simulink library "medusa5h1_stereo"  (R2022b)
settings: Solver=VariableStepAuto  StartTime=0.0  StopTime=10.0  RelTol=1e-3
values from neighbouring files (symbols this model uses):
  MedusaConfig = struct('BandSplitConfig', BandSplitConfig,                            'DRFDPConfig', DRFDPConfig,                            'FRFDPConfig', FRFDPConfig,                            'SurroundConfig', SurroundConfig,                            'MSConfig', MSConfig,                            'PremixConfig', PremixConfig.Stereo,                            'PremixTune', PremixTune.Stereo,               ...(+1303 chars)    [medusa5h1_init.m]
undefined symbols (not defined in the file or in its folder): Config, MedusaBTC, Row, VLSConfig
libraries: TuneVar x25, MedusaDelays x19, FeaturePath x15, RTC x6, MedusaCaeEnable x4, MedusaDrHoligramEq x4, TOP x4, BassManager x2, StateVar x2, TrebleBoost x2, dspstat3 x2, MedusaBandSplit x2
(part 1 of 2)
settings Model: Creator=ud1041536  LastModifiedBy=mp55777
settings SolverCC: AlgebraicLoopSolver=TrustRegion
settings DebuggingCC: UnconnectedInputMsg=warning  UnconnectedOutputMsg=warning  UnconnectedLineMsg=warning  SFMachineParentedDataDiag=warning  ArithmeticOperatorsInVariantConditions=warning
settings ModelReferenceCC: EnableRefExpFcnMdlSchedulingChecks=on
settings SFSimCC: CustomCodeUndefinedFunction=UseInterfaceOnly

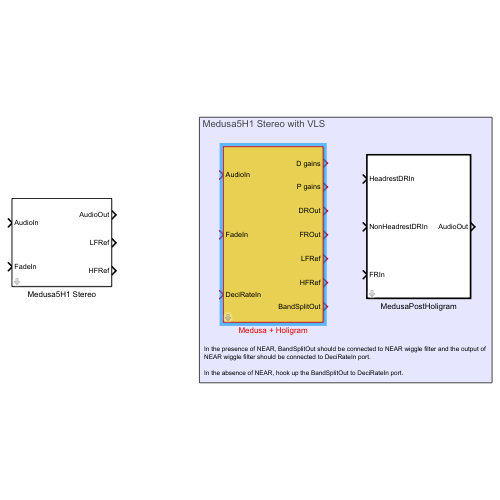
[thumbnail: Simulink's stored preview of the top-level diagram]
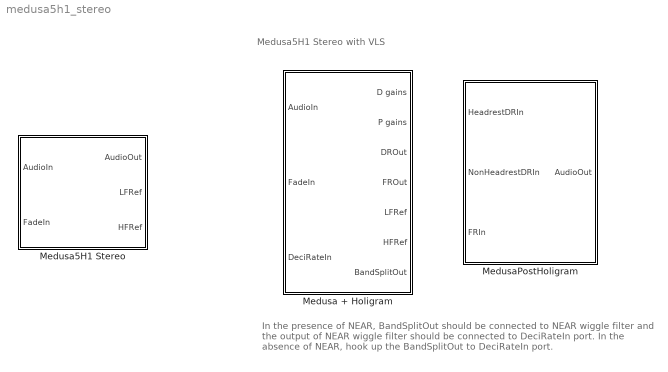
== system medusa5h1_stereo ==
  note: Medusa5H1 Stereo with VLS
  note: In the presence of NEAR, BandSplitOut should be connected to NEAR wiggle filter and the output of
      | NEAR wiggle filter should be connected to DeciRateIn port.
      |
      | In the absence of NEAR, hook up the BandSplitOut to DeciRateIn port.
  Medusa + Holigram : Subsystem  mask{config=MedusaConfig, ConfigBTC=MedusaBTC, vlsConfigStruct=VLSConfig}
      mask prompts: config "Medusa config struct name:"; ConfigBTC "Medusa BTC config struct name:"; vlsConfigStruct "VLS config struct name:"
      mask init:
      | tailCompEQ = config.tailCompEQ;
      | HRDelayConfig = vlsConfigStruct.HeadrestDelayConfig;
      settings: LibrarySourceBlock=medusa5h1_stereo/Medusa + Holigram
  Medusa5H1 Stereo : Subsystem  mask{config=MedusaConfig}
      mask prompts: config "Config struct name:"
      mask init:
      | tailCompEQ = config.tailCompEQ;
      | % delayConfig = config.DelayConfig;
      | 
      | % % Set 2 Medusa parts to be atomic if in Indirect Addressing Mode
      | % isIndirect = CoreIndexMask.IsIndirectAddressing(gcbh);
      | % if isIndirect
      | %     atomicSetting = 'on';
      | % else
      | %     atomicSetting = 'off';
      | % end
      | % p1Name = MaskUtil.SubBlockName(gcbh, 'Medusa5H1 Part 1');
      | % p2Name = MaskUtil.SubBlockName(gcbh, 'Medusa5H1 Part 2');
      | % 
      | % if -1 ~= (getSimulinkBlockHandle(p1Name))
      | %     MaskUtil.safe_setparam(p1Name, 'TreatAsAtomicUnit', atomicSetting);
      | % end
      | % 
      | % if -1 ~= (getSimulinkBlockHandle(p2Name))
      | %     MaskUtil.safe_setparam(p2Name, 'TreatAsAtomicUnit', atomicSetting);
      | % end
  MedusaPostHoligram : Subsystem  TreatAsAtomicUnit=on  mask{config=MedusaConfig}
      mask prompts: config "Config struct name:"
      settings: RTWSystemCode=Nonreusable function  RTWFcnNameOpts=Use subsystem name  RTWFileNameOpts=Use subsystem name  FunctionWithSeparateData=on

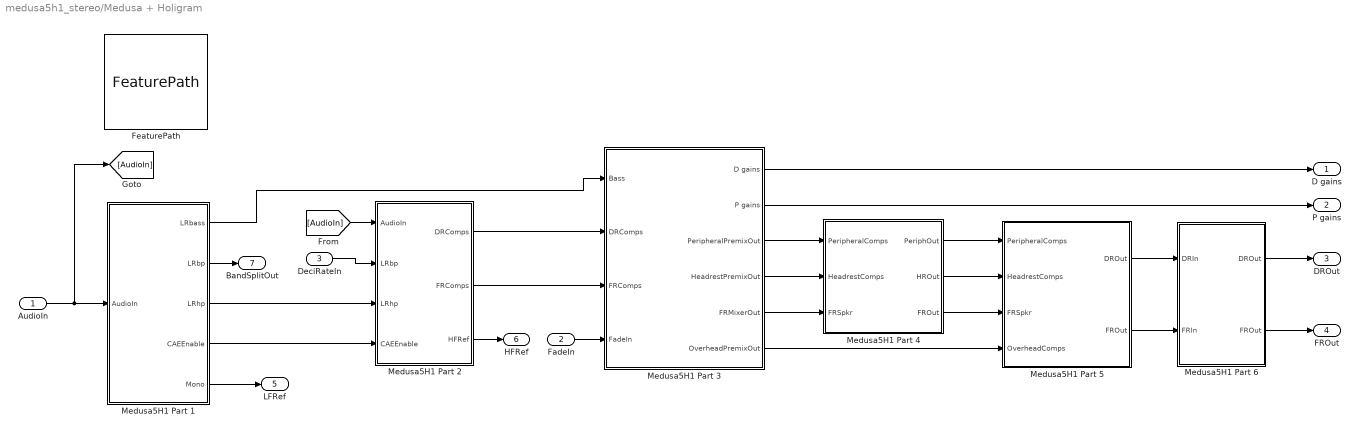
== system medusa5h1_stereo/Medusa + Holigram ==
  AudioIn : Inport
  FadeIn : Inport  Port=2  OutDataTypeStr=single
  DeciRateIn : Inport  Port=3
  FeaturePath : FeaturePath/FeaturePath  FeatureName=Medusa  IsGroup=off  GroupNumber=-1  IsModule=off  TriggerInit=[90 69 205 176]
      settings: SourceProductName=Bose Talaria
  Medusa5H1 Part 1 : Subsystem  TreatAsAtomicUnit=on
      settings: RTWSystemCode=Nonreusable function
  Medusa5H1 Part 2 : Subsystem  TreatAsAtomicUnit=on
      settings: RTWSystemCode=Nonreusable function
  Medusa5H1 Part 3 : Subsystem  TreatAsAtomicUnit=on
      settings: RTWSystemCode=Nonreusable function  FunctionWithSeparateData=on
  Medusa5H1 Part 4 : Subsystem  TreatAsAtomicUnit=on  RTWFcnName=MedusaHoligram  RTWFileName=MedusaHoligram
      settings: RTWSystemCode=Nonreusable function  FunctionWithSeparateData=on
  Medusa5H1 Part 5 : Subsystem  TreatAsAtomicUnit=on
      settings: RTWSystemCode=Nonreusable function  FunctionWithSeparateData=on
  Medusa5H1 Part 6 : Subsystem  TreatAsAtomicUnit=on
      settings: RTWSystemCode=Nonreusable function  FunctionWithSeparateData=on
  D gains : Outport
  P gains : Outport  Port=2
  DROut : Outport  Port=3
  FROut : Outport  Port=4
  LFRef : Outport  Port=5  VectorParamsAs1DForOutWhenUnconnected=off
  HFRef : Outport  Port=6  VectorParamsAs1DForOutWhenUnconnected=off
  BandSplitOut : Outport  Port=7
  wires:
  Medusa5H1 Part 2/2(FRComps) -> Medusa5H1 Part 3/3(FRComps)
  Medusa5H1 Part 2/1(DRComps) -> Medusa5H1 Part 3/2(DRComps)
  FadeIn/1 -> Medusa5H1 Part 3/4(FadeIn)
  AudioIn/1 -> [AudioIn], Medusa5H1 Part 1/1(AudioIn)
  Medusa5H1 Part 1/5(Mono) -> LFRef/1
  Medusa5H1 Part 1/3(LRhp) -> Medusa5H1 Part 2/3(LRhp)
  [AudioIn] -> Medusa5H1 Part 2/1(AudioIn)
  Medusa5H1 Part 1/1(LRbass) -> Medusa5H1 Part 3/1(Bass)
  Medusa5H1 Part 3/2(P gains) -> P gains/1
  Medusa5H1 Part 3/1(D gains) -> D gains/1
  Medusa5H1 Part 6/1(DROut) -> DROut/1
  Medusa5H1 Part 6/2(FROut) -> FROut/1
  Medusa5H1 Part 2/3(HFRef) -> HFRef/1
  Medusa5H1 Part 1/4(CAEEnable) -> Medusa5H1 Part 2/4(CAEEnable)
  Medusa5H1 Part 3/3(PeripheralPremixOut) -> Medusa5H1 Part 4/1(PeripheralComps)
  Medusa5H1 Part 3/4(HeadrestPremixOut) -> Medusa5H1 Part 4/2(HeadrestComps)
  Medusa5H1 Part 3/5(FRMixerOut) -> Medusa5H1 Part 4/3(FRSpkr)
  Medusa5H1 Part 1/2(LRbp) -> BandSplitOut/1
  DeciRateIn/1 -> Medusa5H1 Part 2/2(LRbp)
  Medusa5H1 Part 4/1(PeriphOut) -> Medusa5H1 Part 5/1(PeripheralComps)
  Medusa5H1 Part 4/2(HROut) -> Medusa5H1 Part 5/2(HeadrestComps)
  Medusa5H1 Part 4/3(FROut) -> Medusa5H1 Part 5/3(FRSpkr)
  Medusa5H1 Part 5/1(DROut) -> Medusa5H1 Part 6/1(DRIn)
  Medusa5H1 Part 5/2(FROut) -> Medusa5H1 Part 6/2(FRIn)
  Medusa5H1 Part 3/6(OverheadPremixOut) -> Medusa5H1 Part 5/4(OverheadComps)

== system medusa5h1_stereo/Medusa5H1 Stereo ==
  AudioIn : Inport
  FadeIn : Inport  Port=2  OutDataTypeStr=single
  FeaturePath : FeaturePath/FeaturePath  FeatureName=Medusa  IsGroup=off  GroupNumber=-1  IsModule=off  TriggerInit=[615 344 730 451]
      settings: SourceProductName=Bose Talaria
  Medusa5H1 Part 1 : Subsystem  TreatAsAtomicUnit=on
      settings: RTWSystemCode=Nonreusable function
  Medusa5H1 Part 2 : Subsystem  TreatAsAtomicUnit=on
      settings: RTWSystemCode=Nonreusable function
  Medusa5H1 Part 3 : Subsystem  TreatAsAtomicUnit=on
      settings: RTWSystemCode=Nonreusable function  FunctionWithSeparateData=on
  Medusa5H1 Part 4 : Subsystem  TreatAsAtomicUnit=on
      settings: RTWSystemCode=Nonreusable function  FunctionWithSeparateData=on
  AudioOut : Outport  VectorParamsAs1DForOutWhenUnconnected=off
  LFRef : Outport  Port=2  VectorParamsAs1DForOutWhenUnconnected=off
  HFRef : Outport  Port=3  VectorParamsAs1DForOutWhenUnconnected=off
  wires:
  Medusa5H1 Part 1/1(LRbass) -> Medusa5H1 Part 3/1(Bass)
  Medusa5H1 Part 2/1(DRComps) -> Medusa5H1 Part 3/2(DRComps)
  Medusa5H1 Part 2/2(FRComps) -> Medusa5H1 Part 3/3(FRComps)
  FadeIn/1 -> Medusa5H1 Part 3/4(FadeIn)
  Medusa5H1 Part 1/2(LRbp) -> Medusa5H1 Part 2/2(LRbp)
  Medusa5H1 Part 1/3(LRhp) -> Medusa5H1 Part 2/3(LRhp)
  AudioIn/1 -> [AudioIn], Medusa5H1 Part 1/1(AudioIn)
  [AudioIn] -> Medusa5H1 Part 2/1(AudioIn)
  Medusa5H1 Part 4/1(Out) -> AudioOut/1
  Medusa5H1 Part 3/1(PeripheralPremixOut) -> Medusa5H1 Part 4/1(PeripheralPremixComps)
  Medusa5H1 Part 3/3(FRMixerOut) -> Medusa5H1 Part 4/3(FRSpkrs)
  Medusa5H1 Part 1/5(Mono) -> LFRef/1
  Medusa5H1 Part 2/3(HFRef) -> HFRef/1
  Medusa5H1 Part 1/4(CAEEnable) -> Medusa5H1 Part 2/4(CAEEnable)
  Medusa5H1 Part 3/2(OverheadPremixOut) -> Medusa5H1 Part 4/2(OverheadPremixComps)

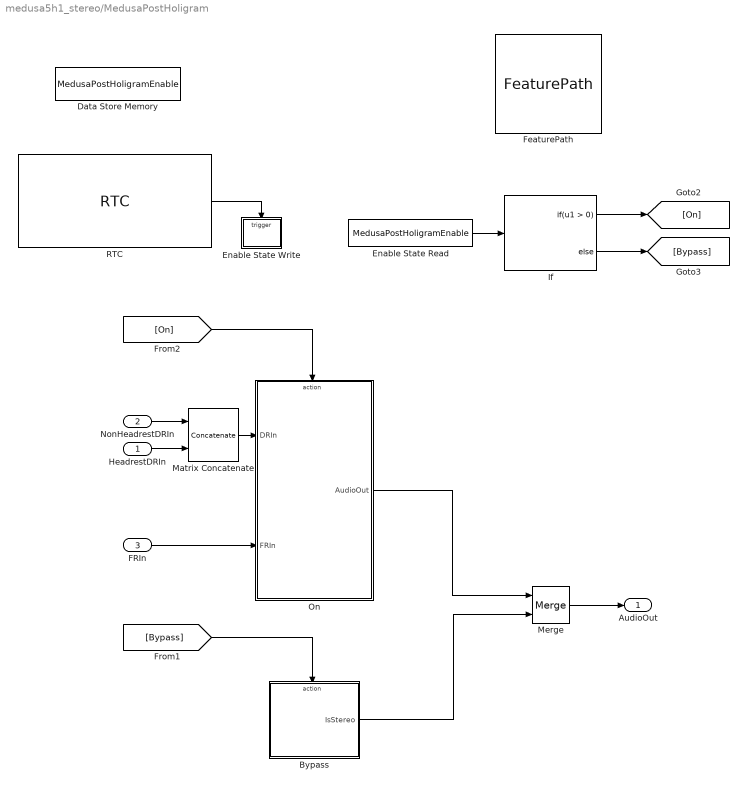
== system medusa5h1_stereo/MedusaPostHoligram ==
  HeadrestDRIn : Inport
  NonHeadrestDRIn : Inport  Port=2
  FRIn : Inport  Port=3
  Bypass : Subsystem
  Data Store Memory : DataStoreMemory  DataStoreName=MedusaPostHoligramEnable  ReadBeforeWriteMsg=warning  WriteAfterWriteMsg=warning  WriteAfterReadMsg=warning  InitialValue=1  ShowAdditionalParam=off  OutDataTypeStr=uint32
  Enable State Read : DataStoreRead  DataStoreName=MedusaPostHoligramEnable  IndexOptions=Index vector (dialog)  Indices=1  OutputSizes=1
  Enable State Write : Subsystem
  FeaturePath : FeaturePath/FeaturePath  FeatureName=Medusa  IsGroup=off  GroupNumber=-1  IsModule=off  TriggerInit=[810 309 925 416]
      settings: SourceProductName=Bose Talaria
  If : If
  Matrix Concatenate : Concatenate  Mode=Multidimensional array  ConcatenateDimension=2
  Merge : Merge  InitialOutput=MedusaConfig.outputDefault
  On : Subsystem
  RTC : RTC/RTC  REQ_Priority=RTC_Mask.NormalPriority  RequestAtInit=off  EnableRequest=on  REQElemType1=int32  REQElemWidth1=1  REQElemInitial1=[]  REQElemType2=uint32  REQElemWidth2=1  REQElemInitial2=[]  REQElemType3=uint32  REQElemWidth3=1  REQElemInitial3=[]  REQElemType4=uint32  REQElemWidth4=1  REQElemInitial4=[]  REQElemType5=uint32  REQElemWidth5=1  REQElemInitial5=[]  REQElemType6=uint32  REQElemWidth6=1  REQElemInitial6=[]  REQElemType7=uint32  REQElemWidth7=1  REQElemInitial7=[]  REQElemType8=uint32  REQElemWidth8=1  REQElemInitial8=[]  REQElemType9=uint32  REQElemWidth9=1  REQElemInitial9=[]  REQElemType10=uint32  REQElemWidth10=1  REQElemInitial10=[]  EnableResponse=on  EnableRSP_StatusIn=off  RSPElemType1=uint32  RSPElemWidth1=1  RSPElemType2=uint32  RSPElemWidth2=1  RSPElemType3=uint32  RSPElemWidth3=1  RSPElemType4=uint32  RSPElemWidth4=1  RSPElemType5=uint32  RSPElemWidth5=1  RSPElemType6=uint32  RSPElemWidth6=1  RSPElemType7=uint32  RSPElemWidth7=1  RSPElemType8=uint32  RSPElemWidth8=1  RSPElemType9=uint32  RSPElemWidth9=1  RSPElemType10=uint32  RSPElemWidth10=1  EnableNotification=off  EnableNTF_PrepTrig=off  NTFElemType1=uint32  NTFElemWidth1=1  NTFElemType2=uint32  NTFElemWidth2=1  NTFElemType3=uint32  NTFElemWidth3=1  NTFElemType4=uint32  NTFElemWidth4=1  NTFElemType5=uint32  NTFElemWidth5=1  NTFElemType6=uint32  NTFElemWidth6=1  NTFElemType7=uint32  NTFElemWidth7=1  NTFElemType8=uint32  NTFElemWidth8=1  NTFElemType9=uint32  NTFElemWidth9=1  NTFElemType10=uint32  NTFElemWidth10=1  MaskMessageName=PostHoligramDisable
      settings: SourceProductName=Bose Talaria
  AudioOut : Outport  VectorParamsAs1DForOutWhenUnconnected=off
  wires:
  FRIn/1 -> On/2(FRIn)
  [Bypass] -> Bypass/Action
  Bypass/1(IsStereo) -> Merge/2
  On/1(AudioOut) -> Merge/1
  Merge/1 -> AudioOut/1
  If/1 -> [On]
  If/2 -> [Bypass]
  Enable State Read/1 -> If/1
  [On] -> On/Action
  RTC/1 -> Enable State Write/Trigger
  Matrix Concatenate/1 -> On/1(DRIn)
  NonHeadrestDRIn/1 -> Matrix Concatenate/1
  HeadrestDRIn/1 -> Matrix Concatenate/2

== system medusa5h1_stereo/Medusa + Holigram/Medusa5H1 Part 1 ==
  AudioIn : Inport
  Bass Manager Stereo : BassManager/MedusaBassManager  Config=ConfigBTC.BassManager
  CAE Treble Boost : Subsystem  Variant=on
  Mean : dspstat3/Mean  run=off  InputProcessing=Columns as channels (frame based)  reset_popup=None  directionMode=Each row  dimension=1  roiEnable=off  roiType=Rectangles  roiPortion=Entire ROI  roiOutput=Individual statistics for each ROI  roiFlag=off  roundingMode=Floor  overflowMode=off  outputDataTypeStr=Inherit: Same as accumulator  outputMin=[]  outputMax=[]  outputLastDataTypeStr=Inherit: Same as accumulator
  Medusa Band Split Stereo : MedusaBandSplit/Medusa Band Split Stereo  configStruct=config.BandSplitConfig
  Partition : FeaturePath/Partition  PartitionNumber=2  TriggerInit=[375 -99 420 -31]
      settings: SourceProductName=Bose Talaria
  Terminator : Terminator
  TuneVar : TuneVar/TuneVar  Description=|  TuneName=SurroundOn  SpecifyMaxSize=off  VariableDim=1 (Row)  MaxSize=[1 1]  TunabilityNumber=1  MinValue=[]  MaxValue=[]  TriggerInit=[235 97 315 133]  MaskValue=ConfigBTC.TuneVarBmSurroundOn
      | General surround control parameter
      | STEREO_MODE = 0
      | SURROUND_PASSTHRU_MODE = 1
      | MEDUSA_2_CHANNEL_MODE = 2
      | MEDUSA_5_1_MODE = 3
      settings: SourceProductName=Bose Talaria
  LRbass : Outport  VectorParamsAs1DForOutWhenUnconnected=off
  LRbp : Outport  Port=2  VectorParamsAs1DForOutWhenUnconnected=off
  LRhp : Outport  Port=3  VectorParamsAs1DForOutWhenUnconnected=off
  CAEEnable : Outport  Port=4
  Mono : Outport  Port=5  VectorParamsAs1DForOutWhenUnconnected=off
  wires:
  Medusa Band Split Stereo/2 -> LRhp/1  "LRtreble"
  Bass Manager Stereo/1 -> LRbass/1  "Lbass, Rbass"
  Medusa Band Split Stereo/1 -> LRbp/1  "LRbp"
  Bass Manager Stereo/2 -> Medusa Band Split Stereo/1
  CAE Treble Boost/1(Out) -> Mean/1, Bass Manager Stereo/1  "L, R"
  Mean/1 -> Mono/1
  AudioIn/1 -> CAE Treble Boost/1(AudioIn)  "L, R"
  CAE Treble Boost/2(CAEEnable) -> CAEEnable/1
  Bass Manager Stereo/3 -> Terminator/1
  TuneVar/1 -> Bass Manager Stereo/2  "SurroundOn"

== system medusa5h1_stereo/Medusa + Holigram/Medusa5H1 Part 2 ==
  AudioIn : Inport  OutDataTypeStr=single
  LRbp : Inport  Port=2
  LRhp : Inport  Port=3
  CAEEnable : Inport  Port=4
  Alignment Delay : Subsystem  TreatAsAtomicUnit=on
      settings: RTWSystemCode=Nonreusable function  FunctionWithSeparateData=on
  Decimated-Rate FDP : MedusaFdp/MedusaFdp  Config=ConfigBTC.DeciRateFdp
  Full-Rate FDP : MedusaFdp/MedusaFdp  Config=ConfigBTC.FullRateFdp
  Mono Detector : MonoDetector/MedusaMonoDetector  Config=ConfigBTC.MonoDetector
  Partition : FeaturePath/Partition  PartitionNumber=3  TriggerInit=[825 236 870 304]
      settings: SourceProductName=Bose Talaria
  SPUM Decay Estimate : MedusaSPUMDecayEst/SPUM Decay Estimate  configStruct=config.FRFDPConfig
  Selector : Selector  NumberOfDimensions=2  InputPortWidth=3  IndexOptions=Select all,Index vector (dialog)  Indices=[1 3],[1,2]  OutputSizes=1,1
  Selector1 : Selector  NumberOfDimensions=2  InputPortWidth=3  IndexOptions=Select all,Index vector (dialog)  Indices=[1 3],[1 2 3 5]  OutputSizes=1,1
  DRComps : Outport  VectorParamsAs1DForOutWhenUnconnected=off
  FRComps : Outport  Port=2  VectorParamsAs1DForOutWhenUnconnected=off
  HFRef : Outport  Port=3
  wires:
  Decimated-Rate FDP/1 -> DRComps/1  "Lo, Ro, Ls, Rs, Limp, Ltail, Rimp, Rtail"
  SPUM Decay Estimate/1 -> Full-Rate FDP/3, Decimated-Rate FDP/3
  Mono Detector/1 -> [isStereo]
  Selector/1 -> Mono Detector/1  "L, R"
  AudioIn/1 -> Selector/1
  LRbp/1 -> Decimated-Rate FDP/1
  LRhp/1 -> Alignment Delay/1(LRhp), SPUM Decay Estimate/1
  [isStereo] -> SPUM Decay Estimate/2
  Full-Rate FDP/1 -> Selector1/1, FRComps/1  "Lo, Ro, Limp, Ltail, Rimp, Rtail"
  Selector1/1 -> HFRef/1  "Lo, Ro, Limp, Rimp"
  CAEEnable/1 -> Decimated-Rate FDP/2, Full-Rate FDP/2
  Alignment Delay/1(LRtreble) -> Full-Rate FDP/1

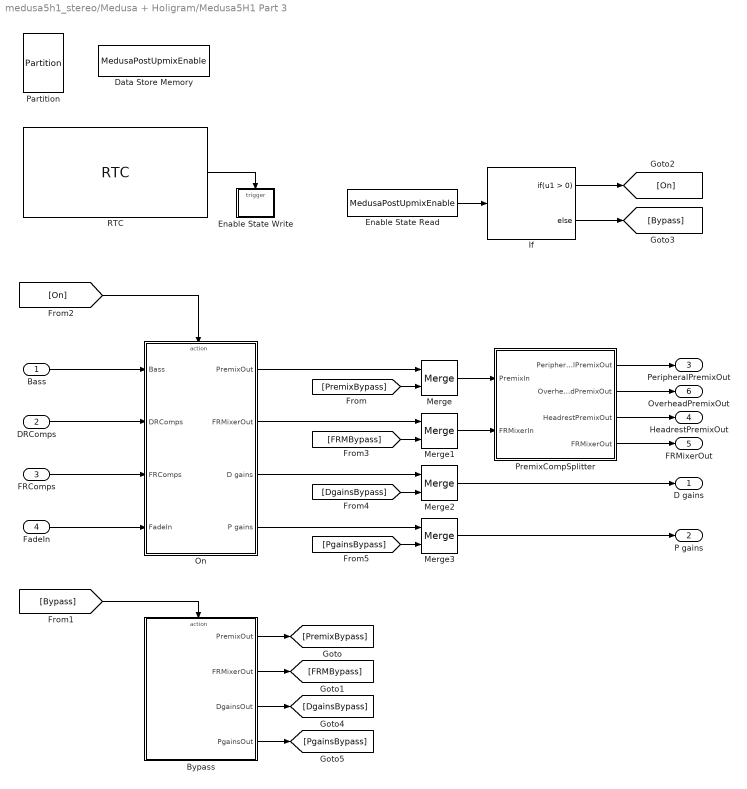
== system medusa5h1_stereo/Medusa + Holigram/Medusa5H1 Part 3 ==
  Bass : Inport
  DRComps : Inport  Port=2
  FRComps : Inport  Port=3
  FadeIn : Inport  Port=4
  Bypass : Subsystem
  Data Store Memory : DataStoreMemory  DataStoreName=MedusaPostUpmixEnable  ReadBeforeWriteMsg=warning  WriteAfterWriteMsg=warning  WriteAfterReadMsg=warning  InitialValue=1  ShowAdditionalParam=off  OutDataTypeStr=uint32
  Enable State Read : DataStoreRead  DataStoreName=MedusaPostUpmixEnable  IndexOptions=Index vector (dialog)  Indices=1  OutputSizes=1
  Enable State Write : Subsystem
  If : If
  Merge : Merge  InitialOutput=zeros(config.HoligramEQConfig.frameSize, config.PremixConfig.NumPremixOut)
  Merge1 : Merge  InitialOutput=ConfigBTC.DefaultFullRateMixerOutput
  Merge2 : Merge  InitialOutput=zeros(config.numVLSGains, 1)
  Merge3 : Merge  InitialOutput=zeros(config.numVLSGains, 1)
  On : Subsystem
  Partition : FeaturePath/Partition  PartitionNumber=5  TriggerInit=[410 331 455 399]
      settings: SourceProductName=Bose Talaria
  PremixCompSplitter : Subsystem
  RTC : RTC/RTC  REQ_Priority=RTC_Mask.NormalPriority  RequestAtInit=off  EnableRequest=on  REQElemType1=int32  REQElemWidth1=1  REQElemInitial1=[]  REQElemType2=uint32  REQElemWidth2=1  REQElemInitial2=[]  REQElemType3=uint32  REQElemWidth3=1  REQElemInitial3=[]  REQElemType4=uint32  REQElemWidth4=1  REQElemInitial4=[]  REQElemType5=uint32  REQElemWidth5=1  REQElemInitial5=[]  REQElemType6=uint32  REQElemWidth6=1  REQElemInitial6=[]  REQElemType7=uint32  REQElemWidth7=1  REQElemInitial7=[]  REQElemType8=uint32  REQElemWidth8=1  REQElemInitial8=[]  REQElemType9=uint32  REQElemWidth9=1  REQElemInitial9=[]  REQElemType10=uint32  REQElemWidth10=1  REQElemInitial10=[]  EnableResponse=on  EnableRSP_StatusIn=off  RSPElemType1=uint32  RSPElemWidth1=1  RSPElemType2=uint32  RSPElemWidth2=1  RSPElemType3=uint32  RSPElemWidth3=1  RSPElemType4=uint32  RSPElemWidth4=1  RSPElemType5=uint32  RSPElemWidth5=1  RSPElemType6=uint32  RSPElemWidth6=1  RSPElemType7=uint32  RSPElemWidth7=1  RSPElemType8=uint32  RSPElemWidth8=1  RSPElemType9=uint32  RSPElemWidth9=1  RSPElemType10=uint32  RSPElemWidth10=1  EnableNotification=off  EnableNTF_PrepTrig=off  NTFElemType1=uint32  NTFElemWidth1=1  NTFElemType2=uint32  NTFElemWidth2=1  NTFElemType3=uint32  NTFElemWidth3=1  NTFElemType4=uint32  NTFElemWidth4=1  NTFElemType5=uint32  NTFElemWidth5=1  NTFElemType6=uint32  NTFElemWidth6=1  NTFElemType7=uint32  NTFElemWidth7=1  NTFElemType8=uint32  NTFElemWidth8=1  NTFElemType9=uint32  NTFElemWidth9=1  NTFElemType10=uint32  NTFElemWidth10=1  MaskMessageName=PostUpmixDisable
      settings: SourceProductName=Bose Talaria
  D gains : Outport
  P gains : Outport  Port=2
  PeripheralPremixOut : Outport  Port=3  VectorParamsAs1DForOutWhenUnconnected=off
  HeadrestPremixOut : Outport  Port=4  VectorParamsAs1DForOutWhenUnconnected=off
  FRMixerOut : Outport  Port=5  VectorParamsAs1DForOutWhenUnconnected=off
  OverheadPremixOut : Outport  Port=6  VectorParamsAs1DForOutWhenUnconnected=off
  wires:
  [PgainsBypass] -> Merge3/2
  [DgainsBypass] -> Merge2/2
  [FRMBypass] -> Merge1/2
  [PremixBypass] -> Merge/2
  Bypass/4(PgainsOut) -> [PgainsBypass]
  Bypass/3(DgainsOut) -> [DgainsBypass]
  Bypass/2(FRMixerOut) -> [FRMBypass]
  Bypass/1(PremixOut) -> [PremixBypass]
  FadeIn/1 -> On/4(FadeIn)
  FRComps/1 -> On/3(FRComps)
  Bass/1 -> On/1(Bass)
  DRComps/1 -> On/2(DRComps)
  [Bypass] -> Bypass/Action
  On/1(PremixOut) -> Merge/1
  If/1 -> [On]
  If/2 -> [Bypass]
  Enable State Read/1 -> If/1
  [On] -> On/Action
  RTC/1 -> Enable State Write/Trigger
  On/2(FRMixerOut) -> Merge1/1
  On/3(D gains) -> Merge2/1
  On/4(P gains) -> Merge3/1
  Merge2/1 -> D gains/1
  Merge3/1 -> P gains/1
  Merge/1 -> PremixCompSplitter/1(PremixIn)
  Merge1/1 -> PremixCompSplitter/2(FRMixerIn)
  PremixCompSplitter/1(PeripheralPremixOut) -> PeripheralPremixOut/1
  PremixCompSplitter/2(OverheadPremixOut) -> OverheadPremixOut/1
  PremixCompSplitter/3(HeadrestPremixOut) -> HeadrestPremixOut/1
  PremixCompSplitter/4(FRMixerOut) -> FRMixerOut/1

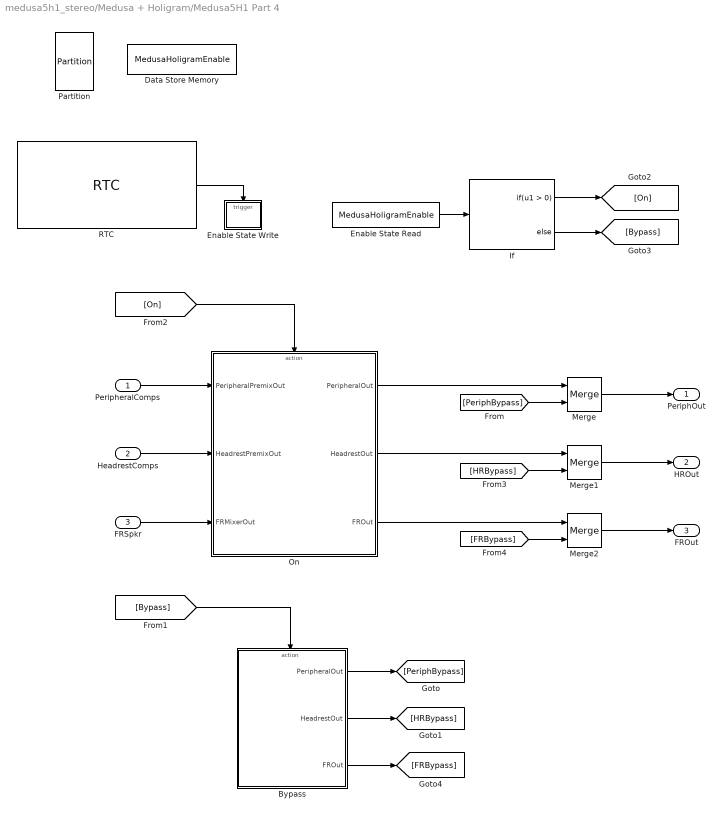
== system medusa5h1_stereo/Medusa + Holigram/Medusa5H1 Part 4 ==
  PeripheralComps : Inport
  HeadrestComps : Inport  Port=2
  FRSpkr : Inport  Port=3
  Bypass : Subsystem
  Data Store Memory : DataStoreMemory  DataStoreName=MedusaHoligramEnable  ReadBeforeWriteMsg=warning  WriteAfterWriteMsg=warning  WriteAfterReadMsg=warning  InitialValue=1  ShowAdditionalParam=off  OutDataTypeStr=uint32
  Enable State Read : DataStoreRead  DataStoreName=MedusaHoligramEnable  IndexOptions=Index vector (dialog)  Indices=1  OutputSizes=1
  Enable State Write : Subsystem
  If : If
  Merge : Merge  InitialOutput=zeros(ConfigBTC.DeciRateFrameSize, ConfigBTC.NumPeripheralChannels)
  Merge1 : Merge  InitialOutput=zeros(ConfigBTC.DeciRateFrameSize, 2*ConfigBTC.NumHeadrestComps)
  Merge2 : Merge  InitialOutput=ConfigBTC.DefaultFullRateMixerOutput
  On : Subsystem
  Partition : FeaturePath/Partition  PartitionNumber=6  TriggerInit=[335 311 380 379]
      settings: SourceProductName=Bose Talaria
  RTC : RTC/RTC  REQ_Priority=RTC_Mask.NormalPriority  RequestAtInit=off  EnableRequest=on  REQElemType1=int32  REQElemWidth1=1  REQElemInitial1=[]  REQElemType2=uint32  REQElemWidth2=1  REQElemInitial2=[]  REQElemType3=uint32  REQElemWidth3=1  REQElemInitial3=[]  REQElemType4=uint32  REQElemWidth4=1  REQElemInitial4=[]  REQElemType5=uint32  REQElemWidth5=1  REQElemInitial5=[]  REQElemType6=uint32  REQElemWidth6=1  REQElemInitial6=[]  REQElemType7=uint32  REQElemWidth7=1  REQElemInitial7=[]  REQElemType8=uint32  REQElemWidth8=1  REQElemInitial8=[]  REQElemType9=uint32  REQElemWidth9=1  REQElemInitial9=[]  REQElemType10=uint32  REQElemWidth10=1  REQElemInitial10=[]  EnableResponse=on  EnableRSP_StatusIn=off  RSPElemType1=uint32  RSPElemWidth1=1  RSPElemType2=uint32  RSPElemWidth2=1  RSPElemType3=uint32  RSPElemWidth3=1  RSPElemType4=uint32  RSPElemWidth4=1  RSPElemType5=uint32  RSPElemWidth5=1  RSPElemType6=uint32  RSPElemWidth6=1  RSPElemType7=uint32  RSPElemWidth7=1  RSPElemType8=uint32  RSPElemWidth8=1  RSPElemType9=uint32  RSPElemWidth9=1  RSPElemType10=uint32  RSPElemWidth10=1  EnableNotification=off  EnableNTF_PrepTrig=off  NTFElemType1=uint32  NTFElemWidth1=1  NTFElemType2=uint32  NTFElemWidth2=1  NTFElemType3=uint32  NTFElemWidth3=1  NTFElemType4=uint32  NTFElemWidth4=1  NTFElemType5=uint32  NTFElemWidth5=1  NTFElemType6=uint32  NTFElemWidth6=1  NTFElemType7=uint32  NTFElemWidth7=1  NTFElemType8=uint32  NTFElemWidth8=1  NTFElemType9=uint32  NTFElemWidth9=1  NTFElemType10=uint32  NTFElemWidth10=1  MaskMessageName=HoligramDisable
      settings: SourceProductName=Bose Talaria
  PeriphOut : Outport  VectorParamsAs1DForOutWhenUnconnected=off
  HROut : Outport  Port=2  VectorParamsAs1DForOutWhenUnconnected=off
  FROut : Outport  Port=3  VectorParamsAs1DForOutWhenUnconnected=off
  wires:
  [HRBypass] -> Merge1/2
  [PeriphBypass] -> Merge/2
  Bypass/2(HeadrestOut) -> [HRBypass]
  Bypass/1(PeripheralOut) -> [PeriphBypass]
  [Bypass] -> Bypass/Action
  On/1(PeripheralOut) -> Merge/1
  Merge/1 -> PeriphOut/1
  If/1 -> [On]
  If/2 -> [Bypass]
  Enable State Read/1 -> If/1
  [On] -> On/Action
  RTC/1 -> Enable State Write/Trigger
  On/2(HeadrestOut) -> Merge1/1
  Merge1/1 -> HROut/1
  HeadrestComps/1 -> On/2(HeadrestPremixOut)
  FRSpkr/1 -> On/3(FRMixerOut)
  PeripheralComps/1 -> On/1(PeripheralPremixOut)
  Bypass/3(FROut) -> [FRBypass]
  Merge2/1 -> FROut/1
  [FRBypass] -> Merge2/2
  On/3(FROut) -> Merge2/1

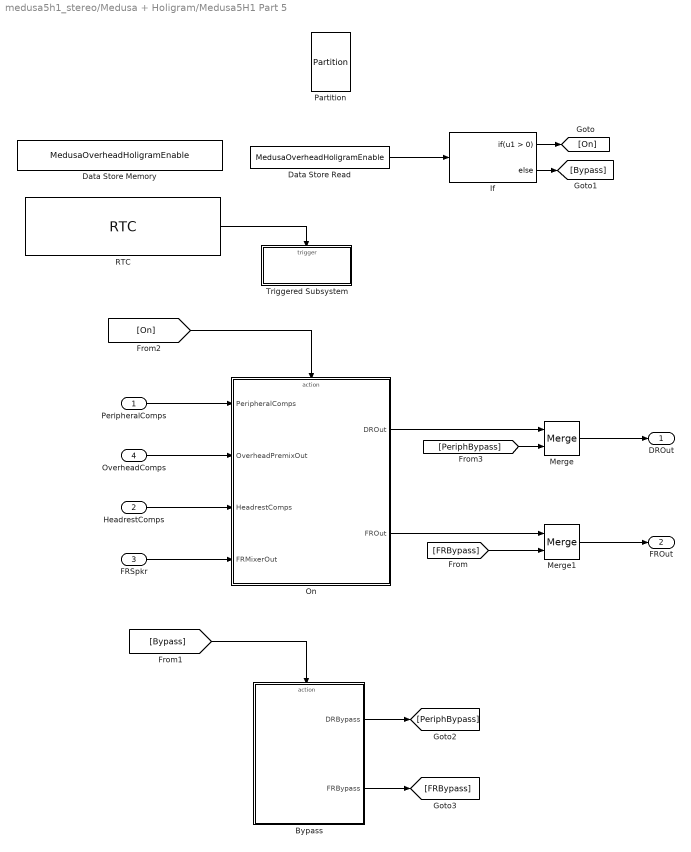
== system medusa5h1_stereo/Medusa + Holigram/Medusa5H1 Part 5 ==
  PeripheralComps : Inport
  HeadrestComps : Inport  Port=2
  FRSpkr : Inport  Port=3
  OverheadComps : Inport  Port=4
  Bypass : Subsystem
  Data Store Memory : DataStoreMemory  DataStoreName=MedusaOverheadHoligramEnable  WriteAfterWriteMsg=warning  InitialValue=1  ShowAdditionalParam=off
  Data Store Read : DataStoreRead  DataStoreName=MedusaOverheadHoligramEnable  IndexOptions=Index vector (dialog)  Indices=1  OutputSizes=1
  If : If
  Merge : Merge
  Merge1 : Merge
  On : Subsystem
  Partition : FeaturePath/Partition  PartitionNumber=7  TriggerInit=[250 -314 295 -246]
      settings: SourceProductName=Bose Talaria
  RTC : RTC/RTC  REQ_Priority=RTC_Mask.NormalPriority  RequestAtInit=off  EnableRequest=on  REQElemType1=uint32  REQElemWidth1=1  REQElemInitial1=[]  REQElemType2=uint32  REQElemWidth2=1  REQElemInitial2=[]  REQElemType3=uint32  REQElemWidth3=1  REQElemInitial3=[]  REQElemType4=uint32  REQElemWidth4=1  REQElemInitial4=[]  REQElemType5=uint32  REQElemWidth5=1  REQElemInitial5=[]  REQElemType6=uint32  REQElemWidth6=1  REQElemInitial6=[]  REQElemType7=uint32  REQElemWidth7=1  REQElemInitial7=[]  REQElemType8=uint32  REQElemWidth8=1  REQElemInitial8=[]  REQElemType9=uint32  REQElemWidth9=1  REQElemInitial9=[]  REQElemType10=uint32  REQElemWidth10=1  REQElemInitial10=[]  EnableResponse=on  EnableRSP_StatusIn=off  RSPElemType1=uint32  RSPElemWidth1=1  RSPElemType2=uint32  RSPElemWidth2=1  RSPElemType3=uint32  RSPElemWidth3=1  RSPElemType4=uint32  RSPElemWidth4=1  RSPElemType5=uint32  RSPElemWidth5=1  RSPElemType6=uint32  RSPElemWidth6=1  RSPElemType7=uint32  RSPElemWidth7=1  RSPElemType8=uint32  RSPElemWidth8=1  RSPElemType9=uint32  RSPElemWidth9=1  RSPElemType10=uint32  RSPElemWidth10=1  EnableNotification=off  EnableNTF_PrepTrig=off  NTFElemType1=uint32  NTFElemWidth1=1  NTFElemType2=uint32  NTFElemWidth2=1  NTFElemType3=uint32  NTFElemWidth3=1  NTFElemType4=uint32  NTFElemWidth4=1  NTFElemType5=uint32  NTFElemWidth5=1  NTFElemType6=uint32  NTFElemWidth6=1  NTFElemType7=uint32  NTFElemWidth7=1  NTFElemType8=uint32  NTFElemWidth8=1  NTFElemType9=uint32  NTFElemWidth9=1  NTFElemType10=uint32  NTFElemWidth10=1  MaskMessageName=OverheadHoligramDisable
      settings: SourceProductName=Bose Talaria
  Triggered Subsystem : Subsystem  TreatAsAtomicUnit=on
  DROut : Outport
  FROut : Outport  Port=2
  wires:
  RTC/1 -> Triggered Subsystem/Trigger
  Data Store Read/1 -> If/1
  If/1 -> [On]
  If/2 -> [Bypass]
  Bypass/2(FRBypass) -> [FRBypass]
  Bypass/1(DRBypass) -> [PeriphBypass]
  [Bypass] -> Bypass/Action
  [On] -> On/Action
  OverheadComps/1 -> On/2(OverheadPremixOut)
  FRSpkr/1 -> On/4(FRMixerOut)
  HeadrestComps/1 -> On/3(HeadrestComps)
  PeripheralComps/1 -> On/1(PeripheralComps)
  On/1(DROut) -> Merge/1
  Merge/1 -> DROut/1
  On/2(FROut) -> Merge1/1
  Merge1/1 -> FROut/1
  [FRBypass] -> Merge1/2
  [PeriphBypass] -> Merge/2

== system medusa5h1_stereo/Medusa + Holigram/Medusa5H1 Part 6 ==
  DRIn : Inport
  FRIn : Inport  Port=2
  DR Speaker and HRComps Delay : MedusaDelays/MedusaTunableDelay  Config=ConfigBTC.DeciRateSpeakerDelay
  FR Speaker Delay : MedusaDelays/MedusaTunableDelay  Config=ConfigBTC.FullRateSpeakerDelay
  Partition : FeaturePath/Partition  PartitionNumber=8  TriggerInit=[1360 586 1405 654]
      settings: SourceProductName=Bose Talaria
  Speaker Delay Tune : Subsystem
  DROut : Outport  VectorParamsAs1DForOutWhenUnconnected=off
  FROut : Outport  Port=2  VectorParamsAs1DForOutWhenUnconnected=off
  wires:
  DRIn/1 -> DR Speaker and HRComps Delay/1
  FRIn/1 -> FR Speaker Delay/1
  FR Speaker Delay/1 -> FROut/1
  [FRSpeakerDelay] -> FR Speaker Delay/2
  Speaker Delay Tune/1(DRSpeakerDelay) -> [DRSpeakerDelay]
  [DRSpeakerDelay] -> DR Speaker and HRComps Delay/2
  Speaker Delay Tune/2(FRSpeakerDelay) -> [FRSpeakerDelay]
  DR Speaker and HRComps Delay/1 -> DROut/1

== system medusa5h1_stereo/Medusa5H1 Stereo/Medusa5H1 Part 1 ==
  AudioIn : Inport
  Bass Manager Stereo : BassManager/MedusaBassManagerStereo  Config=Config.BassManager
  CAE Treble Boost : Subsystem  Variant=on
  Mean : dspstat3/Mean  run=off  InputProcessing=Columns as channels (frame based)  reset_popup=None  directionMode=Each row  dimension=1  roiEnable=off  roiType=Rectangles  roiPortion=Entire ROI  roiOutput=Individual statistics for each ROI  roiFlag=off  roundingMode=Floor  overflowMode=off  outputDataTypeStr=Inherit: Same as accumulator  outputMin=[]  outputMax=[]  outputLastDataTypeStr=Inherit: Same as accumulator
  Medusa Band Split Stereo : MedusaBandSplit/Medusa Band Split Stereo  configStruct=config.BandSplitConfig
  Partition : FeaturePath/Partition  PartitionNumber=2  TriggerInit=[390 -99 435 -31]
      settings: SourceProductName=Bose Talaria
  Selector1 : Selector  NumberOfDimensions=2  InputPortWidth=3  IndexOptions=Select all,Index vector (dialog)  Indices=[1 3],1:2  OutputSizes=1,1
  LRbass : Outport  VectorParamsAs1DForOutWhenUnconnected=off
  LRbp : Outport  Port=2  VectorParamsAs1DForOutWhenUnconnected=off
  LRhp : Outport  Port=3  VectorParamsAs1DForOutWhenUnconnected=off
  CAEEnable : Outport  Port=4
  Mono : Outport  Port=5  VectorParamsAs1DForOutWhenUnconnected=off
  wires:
  Medusa Band Split Stereo/2 -> LRhp/1  "LRtreble"
  AudioIn/1 -> Selector1/1
  Bass Manager Stereo/1 -> LRbass/1  "Lbass, Rbass"
  Medusa Band Split Stereo/1 -> LRbp/1  "LRbp"
  Bass Manager Stereo/2 -> Medusa Band Split Stereo/1
  Mean/1 -> Mono/1
  CAE Treble Boost/1(Out) -> Bass Manager Stereo/1
  CAE Treble Boost/2(CAEEnable) -> CAEEnable/1
  Selector1/1 -> CAE Treble Boost/1(AudioIn), Mean/1  "L, R"

== system medusa5h1_stereo/Medusa5H1 Stereo/Medusa5H1 Part 2 ==
  AudioIn : Inport  OutDataTypeStr=single
  LRbp : Inport  Port=2
  LRhp : Inport  Port=3
  CAEEnable : Inport  Port=4
  Alignment Delay : Subsystem  TreatAsAtomicUnit=on
      settings: RTWSystemCode=Nonreusable function  FunctionWithSeparateData=on
  Decimated-Rate FDP : MedusaFDP/Decimated-Rate  FeatureName=DeciRate  configStruct=config.DRFDPConfig
  Full-Rate FDP : MedusaFullRateFDP/Full-Rate  FeatureName=FullRate  configStruct=config.FRFDPConfig
  Mono Detector : MonoDetector/MedusaMonoDetector  Config=Config.MonoDetector
  Partition : FeaturePath/Partition  PartitionNumber=3  TriggerInit=[820 236 865 304]
      settings: SourceProductName=Bose Talaria
  SPUM Decay Estimate : MedusaSPUMDecayEst/SPUM Decay Estimate  configStruct=config.FRFDPConfig
  Selector : Selector  NumberOfDimensions=2  InputPortWidth=3  IndexOptions=Select all,Index vector (dialog)  Indices=[1 3],[1,2]  OutputSizes=1,1
  Selector1 : Selector  NumberOfDimensions=2  InputPortWidth=3  IndexOptions=Select all,Index vector (dialog)  Indices=[1 3],[1 2 3 5]  OutputSizes=1,1
  DRComps : Outport  VectorParamsAs1DForOutWhenUnconnected=off
  FRComps : Outport  Port=2  VectorParamsAs1DForOutWhenUnconnected=off
  HFRef : Outport  Port=3
  wires:
  Full-Rate FDP/1 -> Selector1/1, FRComps/1  "Lo, Ro, Limp, Ltail, Rimp, Rtail"
  Decimated-Rate FDP/1 -> DRComps/1  "Lo, Ro, Ls, Rs, Limp, Ltail, Rimp, Rtail"
  SPUM Decay Estimate/1 -> Full-Rate FDP/3, Decimated-Rate FDP/3
  CAEEnable/1 -> Full-Rate FDP/2, Decimated-Rate FDP/2
  Mono Detector/1 -> [isStereo]
  Selector/1 -> Mono Detector/1  "L, R"
  AudioIn/1 -> Selector/1
  LRbp/1 -> Decimated-Rate FDP/1
  LRhp/1 -> Alignment Delay/1(LRhp), SPUM Decay Estimate/1
  [isStereo] -> SPUM Decay Estimate/2
  Selector1/1 -> HFRef/1  "Lo, Ro, Limp, Rimp"
  Alignment Delay/1(LRtreble) -> Full-Rate FDP/1

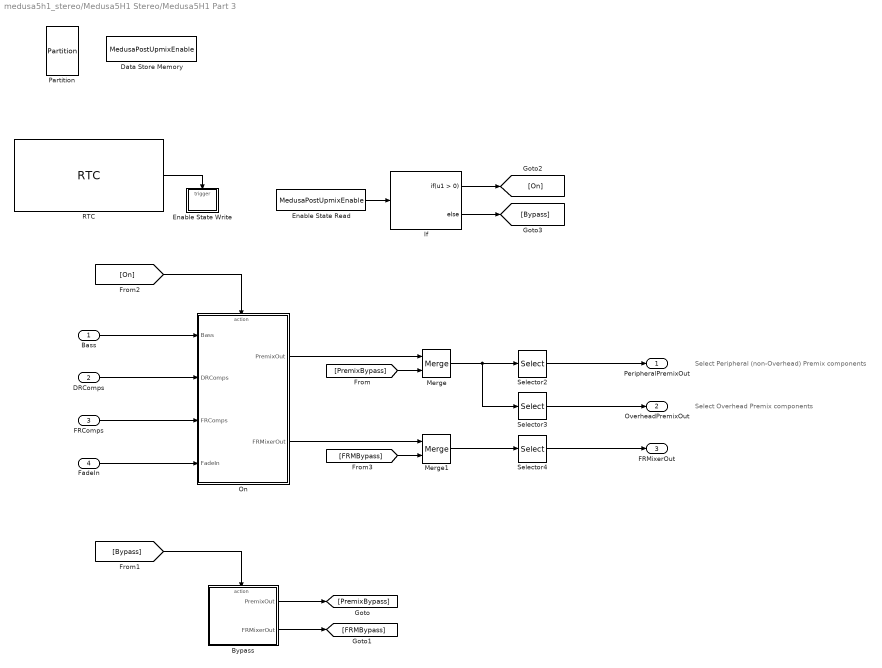
== system medusa5h1_stereo/Medusa5H1 Stereo/Medusa5H1 Part 3 ==
  note: Select Peripheral (non-Overhead) Premix components
  note: Select Overhead Premix components
  Bass : Inport
  DRComps : Inport  Port=2
  FRComps : Inport  Port=3
  FadeIn : Inport  Port=4
  Bypass : Subsystem
  Data Store Memory : DataStoreMemory  DataStoreName=MedusaPostUpmixEnable  ReadBeforeWriteMsg=warning  WriteAfterWriteMsg=warning  WriteAfterReadMsg=warning  InitialValue=1  ShowAdditionalParam=off  OutDataTypeStr=uint32
  Enable State Read : DataStoreRead  DataStoreName=MedusaPostUpmixEnable  IndexOptions=Index vector (dialog)  Indices=1  OutputSizes=1
  Enable State Write : Subsystem
  If : If
  Merge : Merge  InitialOutput=zeros(config.PremixConfig.frame_size, config.PremixConfig.NumPremixOut)
  Merge1 : Merge  InitialOutput=Config.DefaultFullRateMixerOutput
  On : Subsystem
  Partition : FeaturePath/Partition  PartitionNumber=5  TriggerInit=[335 281 380 349]
      settings: SourceProductName=Bose Talaria
  RTC : RTC/RTC  REQ_Priority=RTC_Mask.NormalPriority  RequestAtInit=off  EnableRequest=on  REQElemType1=int32  REQElemWidth1=1  REQElemInitial1=[]  REQElemType2=uint32  REQElemWidth2=1  REQElemInitial2=[]  REQElemType3=uint32  REQElemWidth3=1  REQElemInitial3=[]  REQElemType4=uint32  REQElemWidth4=1  REQElemInitial4=[]  REQElemType5=uint32  REQElemWidth5=1  REQElemInitial5=[]  REQElemType6=uint32  REQElemWidth6=1  REQElemInitial6=[]  REQElemType7=uint32  REQElemWidth7=1  REQElemInitial7=[]  REQElemType8=uint32  REQElemWidth8=1  REQElemInitial8=[]  REQElemType9=uint32  REQElemWidth9=1  REQElemInitial9=[]  REQElemType10=uint32  REQElemWidth10=1  REQElemInitial10=[]  EnableResponse=on  EnableRSP_StatusIn=off  RSPElemType1=uint32  RSPElemWidth1=1  RSPElemType2=uint32  RSPElemWidth2=1  RSPElemType3=uint32  RSPElemWidth3=1  RSPElemType4=uint32  RSPElemWidth4=1  RSPElemType5=uint32  RSPElemWidth5=1  RSPElemType6=uint32  RSPElemWidth6=1  RSPElemType7=uint32  RSPElemWidth7=1  RSPElemType8=uint32  RSPElemWidth8=1  RSPElemType9=uint32  RSPElemWidth9=1  RSPElemType10=uint32  RSPElemWidth10=1  EnableNotification=off  EnableNTF_PrepTrig=off  NTFElemType1=uint32  NTFElemWidth1=1  NTFElemType2=uint32  NTFElemWidth2=1  NTFElemType3=uint32  NTFElemWidth3=1  NTFElemType4=uint32  NTFElemWidth4=1  NTFElemType5=uint32  NTFElemWidth5=1  NTFElemType6=uint32  NTFElemWidth6=1  NTFElemType7=uint32  NTFElemWidth7=1  NTFElemType8=uint32  NTFElemWidth8=1  NTFElemType9=uint32  NTFElemWidth9=1  NTFElemType10=uint32  NTFElemWidth10=1  MaskMessageName=PostUpmixDisable
      settings: SourceProductName=Bose Talaria
  Selector2 : Selector  NumberOfDimensions=2  InputPortWidth=3  IndexOptions=Select all,Index vector (dialog)  Indices=[1 3],config.PeripheralIdx  OutputSizes=1,1
  Selector3 : Selector  NumberOfDimensions=2  InputPortWidth=3  IndexOptions=Select all,Index vector (dialog)  Indices=[1 3],config.OverheadIdx  OutputSizes=1,1
  Selector4 : Selector  NumberOfDimensions=2  InputPortWidth=3  IndexOptions=Select all,Index vector (dialog)  Indices=[1 3],config.FRMOutputIdx  OutputSizes=1,1
  PeripheralPremixOut : Outport  VectorParamsAs1DForOutWhenUnconnected=off
  OverheadPremixOut : Outport  Port=2  VectorParamsAs1DForOutWhenUnconnected=off
  FRMixerOut : Outport  Port=3  VectorParamsAs1DForOutWhenUnconnected=off
  wires:
  FadeIn/1 -> On/4(FadeIn)
  FRComps/1 -> On/3(FRComps)
  Bass/1 -> On/1(Bass)
  DRComps/1 -> On/2(DRComps)
  [Bypass] -> Bypass/Action
  On/1(PremixOut) -> Merge/1
  If/1 -> [On]
  If/2 -> [Bypass]
  Enable State Read/1 -> If/1
  [On] -> On/Action
  RTC/1 -> Enable State Write/Trigger
  On/2(FRMixerOut) -> Merge1/1
  Merge1/1 -> Selector4/1
  Merge/1 -> Selector3/1, Selector2/1
  Selector2/1 -> PeripheralPremixOut/1
  Selector3/1 -> OverheadPremixOut/1
  Selector4/1 -> FRMixerOut/1
  [PremixBypass] -> Merge/2
  [FRMBypass] -> Merge1/2
  Bypass/1(PremixOut) -> [PremixBypass]
  Bypass/2(FRMixerOut) -> [FRMBypass]

== system medusa5h1_stereo/Medusa5H1 Stereo/Medusa5H1 Part 4 ==
  PeripheralPremixComps : Inport
  OverheadPremixComps : Inport  Port=2
  FRSpkrs : Inport  Port=3
  Bypass : Subsystem
  Data Store Memory : DataStoreMemory  DataStoreName=MedusaHoligramEnable  ReadBeforeWriteMsg=warning  WriteAfterWriteMsg=warning  WriteAfterReadMsg=warning  InitialValue=1  ShowAdditionalParam=off  OutDataTypeStr=uint32
  Enable State Read : DataStoreRead  DataStoreName=MedusaHoligramEnable  IndexOptions=Index vector (dialog)  Indices=1  OutputSizes=1
  Enable State Write : Subsystem
  If : If
  Merge : Merge  InitialOutput=MedusaConfig.outputDefault
  On : Subsystem
  Partition : FeaturePath/Partition  PartitionNumber=6  TriggerInit=[335 281 380 349]
      settings: SourceProductName=Bose Talaria
  RTC : RTC/RTC  REQ_Priority=RTC_Mask.NormalPriority  RequestAtInit=off  EnableRequest=on  REQElemType1=int32  REQElemWidth1=1  REQElemInitial1=[]  REQElemType2=uint32  REQElemWidth2=1  REQElemInitial2=[]  REQElemType3=uint32  REQElemWidth3=1  REQElemInitial3=[]  REQElemType4=uint32  REQElemWidth4=1  REQElemInitial4=[]  REQElemType5=uint32  REQElemWidth5=1  REQElemInitial5=[]  REQElemType6=uint32  REQElemWidth6=1  REQElemInitial6=[]  REQElemType7=uint32  REQElemWidth7=1  REQElemInitial7=[]  REQElemType8=uint32  REQElemWidth8=1  REQElemInitial8=[]  REQElemType9=uint32  REQElemWidth9=1  REQElemInitial9=[]  REQElemType10=uint32  REQElemWidth10=1  REQElemInitial10=[]  EnableResponse=on  EnableRSP_StatusIn=off  RSPElemType1=uint32  RSPElemWidth1=1  RSPElemType2=uint32  RSPElemWidth2=1  RSPElemType3=uint32  RSPElemWidth3=1  RSPElemType4=uint32  RSPElemWidth4=1  RSPElemType5=uint32  RSPElemWidth5=1  RSPElemType6=uint32  RSPElemWidth6=1  RSPElemType7=uint32  RSPElemWidth7=1  RSPElemType8=uint32  RSPElemWidth8=1  RSPElemType9=uint32  RSPElemWidth9=1  RSPElemType10=uint32  RSPElemWidth10=1  EnableNotification=off  EnableNTF_PrepTrig=off  NTFElemType1=uint32  NTFElemWidth1=1  NTFElemType2=uint32  NTFElemWidth2=1  NTFElemType3=uint32  NTFElemWidth3=1  NTFElemType4=uint32  NTFElemWidth4=1  NTFElemType5=uint32  NTFElemWidth5=1  NTFElemType6=uint32  NTFElemWidth6=1  NTFElemType7=uint32  NTFElemWidth7=1  NTFElemType8=uint32  NTFElemWidth8=1  NTFElemType9=uint32  NTFElemWidth9=1  NTFElemType10=uint32  NTFElemWidth10=1  MaskMessageName=HoligramDisable
      settings: SourceProductName=Bose Talaria
  Out : Outport  VectorParamsAs1DForOutWhenUnconnected=off
  wires:
  PeripheralPremixComps/1 -> On/1(PeripheralPremixOut)
  FRSpkrs/1 -> On/3(FRMixerOut)
  [Bypass] -> Bypass/Action
  Bypass/1(IsStereo) -> Merge/2
  On/1(AudioOut) -> Merge/1
  Merge/1 -> Out/1
  If/1 -> [On]
  If/2 -> [Bypass]
  Enable State Read/1 -> If/1
  [On] -> On/Action
  RTC/1 -> Enable State Write/Trigger
  OverheadPremixComps/1 -> On/2(OverheadPremixOut)

== system medusa5h1_stereo/MedusaPostHoligram/Bypass ==
  Action Port : ActionPort
  Constant : Constant  Value=MedusaConfig.outputDefault  OutDataTypeStr=single
  IsStereo : Outport  VectorParamsAs1DForOutWhenUnconnected=off
  wires:
  Constant/1 -> IsStereo/1

== system medusa5h1_stereo/MedusaPostHoligram/Enable State Write ==
  Trigger : TriggerPort  TriggerType=function-call  VariantControl=Variant  PortDimensions=1
  Constant : Constant  Value=0  OutDataTypeStr=uint32
  Data Store Write : DataStoreWrite  DataStoreName=MedusaPostHoligramEnable  IndexOptions=Index vector (dialog)  Indices=1  OutputSizes=1
  wires:
  Constant/1 -> Data Store Write/1

== system medusa5h1_stereo/MedusaPostHoligram/On ==
  DRIn : Inport  OutDataTypeStr=single
  FRIn : Inport  Port=2  OutDataTypeStr=single
  Action Port : ActionPort
  Add : Sum
  Constant : Constant  Value=config.BandSplitConfig.PostHoligramFirUp.CoeffsTarget
  MedusaFirUp : FirUp/FirUp  Config=config.BandSplitConfig.PostHoligramFirUp
      settings: SourceProductName=Bose Blocklib
  Router : MATLAB Function  TreatAsAtomicUnit=on
  TuneTOP1 : TuneVar/TuneTOP  TriggerInit=[2170 702 2340 758]  TopName=RoutingMap  TuneName=RoutingMap  DataTypeOut=single  TunabilityNumber=1  MinValue=[]  MaxValue=[]  BankNumber=0  PreOverlay=false  PostOverlay=false  UseSameName=on  MaskValue=config.routingMapDefault
      settings: SourceProductName=Bose Talaria
  AudioOut : Outport  VectorParamsAs1DForOutWhenUnconnected=off
  wires:
  DRIn/1 -> MedusaFirUp/1
  Add/1 -> Router/1(u)
  FRIn/1 -> Add/2
  TuneTOP1/1 -> Router/2(routingMap)
  Router/1(y) -> AudioOut/1
  MedusaFirUp/1 -> Add/1
  Constant/1 -> MedusaFirUp/2

== system medusa5h1_stereo/Medusa + Holigram/Medusa5H1 Part 1/CAE Treble Boost ==
  note: 1) Add Subsystem or Model blocks as valid variant choices.
      | 2) You cannot connect blocks at this level. At simulation, connectivity is automatically
      | determined, based on the active variant and port name matching.
  AudioIn : Inport
  Audio Passthrough : Subsystem  VariantControl=sys_defs.include_compressed_audio_enhancement == 0
  CAE Treble Boost : Subsystem  VariantControl=sys_defs.include_compressed_audio_enhancement == 1
  Out : Outport
  CAEEnable : Outport  Port=2

== system medusa5h1_stereo/Medusa + Holigram/Medusa5H1 Part 2/Alignment Delay ==
  LRhp : Inport
  Full-rate Alignment Delay Translation : MedusaDelays/MedusaFullRateAlignmentDelayTranslation  Config=ConfigBTC.TrebleDelayTranslation
  Treble Delay : MedusaDelays/MedusaAlignmentDelay  Config=ConfigBTC.TrebleDelay
  Tune Variable1 : TuneVar/TuneVar  TuneName=DeciRateNearWiggleFilterDelaySamples  SpecifyMaxSize=off  VariableDim=1 (Row)  MaxSize=[1 1]  TunabilityNumber=1  MinValue=[]  MaxValue=[]  TriggerInit=[-15 450 150 500]  MaskValue=ConfigBTC.AlignmentDelayTranslation.DefaultTuning.DeciRateNearWiggleDelay
      settings: SourceProductName=Bose Talaria
  Tune Variable4 : TuneVar/TuneVar  TuneName=DeciRateWiggleFilterDelaySamples  SpecifyMaxSize=off  VariableDim=1 (Row)  MaxSize=[1 1]  TunabilityNumber=1  MinValue=[]  MaxValue=[]  TriggerInit=[-15 385 150 435]  MaskValue=ConfigBTC.AlignmentDelayTranslation.DefaultTuning.DeciRateWiggleDelay
      settings: SourceProductName=Bose Talaria
  Tune Variable5 : TuneVar/TuneVar  TuneName=HoligramFilterAlignmentDelaySamples  SpecifyMaxSize=off  VariableDim=1 (Row)  MaxSize=[1 1]  TunabilityNumber=1  MinValue=[]  MaxValue=[]  TriggerInit=[-15 515 150 565]  MaskValue=ConfigBTC.TrebleDelayTranslation.DefaultTuning.HoligramDelay
      settings: SourceProductName=Bose Talaria
  LRtreble : Outport
  wires:
  Treble Delay/1 -> LRtreble/1  "LRtreble"
  [TrebleDelay] -> Treble Delay/2
  Full-rate Alignment Delay Translation/1 -> [TrebleDelay]
  Tune Variable4/1 -> Full-rate Alignment Delay Translation/1  "DeciRateWiggleFilterDelaySamples"
  LRhp/1 -> Treble Delay/1
  Tune Variable5/1 -> Full-rate Alignment Delay Translation/3  "HoligramFilterAlignmentDelaySamples"
  Tune Variable1/1 -> Full-rate Alignment Delay Translation/2  "DeciRateNearWiggleFilterDelaySamples"

== system medusa5h1_stereo/Medusa + Holigram/Medusa5H1 Part 3/Bypass ==
  Action Port : ActionPort
  Constant : Constant  Value=zeros(config.HoligramEQConfig.frameSize, config.PremixConfig.NumPremixOut)  OutDataTypeStr=single
  Constant1 : Constant  Value=ConfigBTC.DefaultFullRateMixerOutput  OutDataTypeStr=single
  Constant2 : Constant  Value=zeros(config.numVLSGains, 1)  OutDataTypeStr=single
  Constant3 : Constant  Value=zeros(config.numVLSGains, 1)  OutDataTypeStr=single
  PremixOut : Outport  VectorParamsAs1DForOutWhenUnconnected=off
  FRMixerOut : Outport  Port=2  VectorParamsAs1DForOutWhenUnconnected=off
  DgainsOut : Outport  Port=3  VectorParamsAs1DForOutWhenUnconnected=off
  PgainsOut : Outport  Port=4  VectorParamsAs1DForOutWhenUnconnected=off
  wires:
  Constant/1 -> PremixOut/1
  Constant1/1 -> FRMixerOut/1
  Constant3/1 -> PgainsOut/1
  Constant2/1 -> DgainsOut/1

== system medusa5h1_stereo/Medusa + Holigram/Medusa5H1 Part 3/Enable State Write ==
  Trigger : TriggerPort  TriggerType=function-call  VariantControl=Variant  PortDimensions=1
  Constant : Constant  Value=0  OutDataTypeStr=uint32
  Data Store Write : DataStoreWrite  DataStoreName=MedusaPostUpmixEnable  IndexOptions=Index vector (dialog)  Indices=1  OutputSizes=1
  wires:
  Constant/1 -> Data Store Write/1

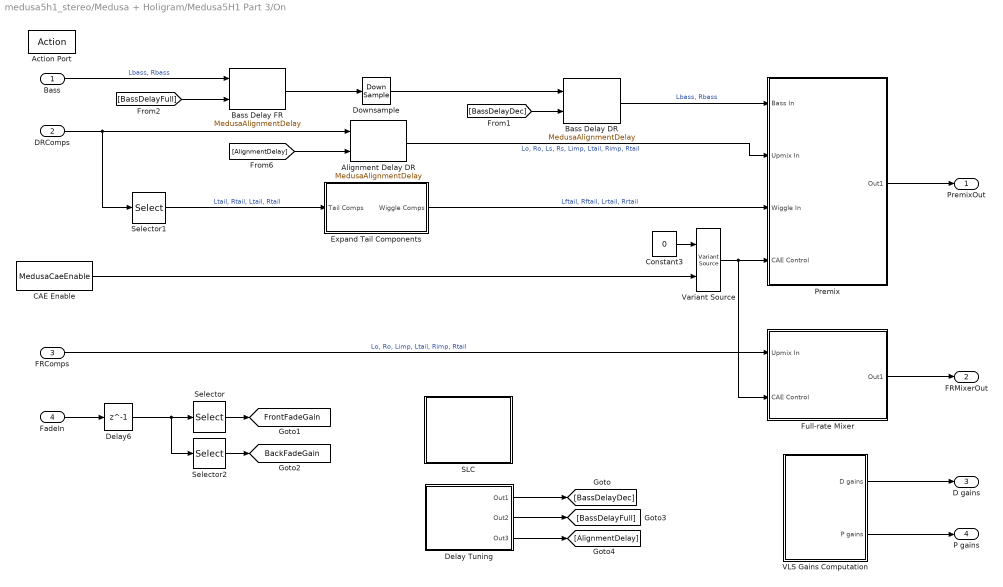
== system medusa5h1_stereo/Medusa + Holigram/Medusa5H1 Part 3/On ==
  Bass : Inport  OutDataTypeStr=single
  DRComps : Inport  Port=2  OutDataTypeStr=single
  FRComps : Inport  Port=3  OutDataTypeStr=single
  FadeIn : Inport  Port=4  OutDataTypeStr=single
  Action Port : ActionPort
  Alignment Delay DR : MedusaDelays/MedusaAlignmentDelay  Config=ConfigBTC.MidrangeDelay
  Bass Delay DR : MedusaDelays/MedusaAlignmentDelay  Config=ConfigBTC.DeciRateBassDelay
  Bass Delay FR : MedusaDelays/MedusaAlignmentDelay  Config=ConfigBTC.FullRateBassDelay
  CAE Enable : MedusaCaeEnable/MedusaCaeEnable  Config=ConfigBTC.PremixCaeEnable  MaskMessageName=PremixCAEEnable
  Constant3 : Constant  Value=0  OutDataTypeStr=int32  SampleTime=-1
  Delay Tuning : Subsystem
  Delay6 : Delay  DelayLength=1
  Downsample : DownSample  N=4
  Expand Tail Components : Subsystem  TreatAsAtomicUnit=on  RTWFileName=MedusaExpandTailComps
      settings: RTWSystemCode=Nonreusable function  RTWFileNameOpts=User specified  FunctionWithSeparateData=on
  Full-rate Mixer : Subsystem
  Premix : Subsystem
  SLC : Subsystem
  Selector : Selector  NumberOfDimensions=2  InputPortWidth=2  IndexOptions=Index vector (dialog),Index vector (dialog)  Indices=1,1  OutputSizes=1,1
  Selector1 : Selector  NumberOfDimensions=2  InputPortWidth=3  IndexOptions=Select all,Index vector (dialog)  Indices=[1 3],[6 8 6 8]  OutputSizes=1,1
  Selector2 : Selector  NumberOfDimensions=2  InputPortWidth=2  IndexOptions=Index vector (dialog),Index vector (dialog)  Indices=1,2  OutputSizes=1,1
  VLS Gains Computation : Subsystem
  Variant Source : VariantSource
  PremixOut : Outport  VectorParamsAs1DForOutWhenUnconnected=off
  FRMixerOut : Outport  Port=2  VectorParamsAs1DForOutWhenUnconnected=off
  D gains : Outport  Port=3
  P gains : Outport  Port=4
  tag scope: BackFadeGain=global, FrontFadeGain=global
  wires:
  Selector/1 -> [FrontFadeGain]
  Delay6/1 -> Selector/1, Selector2/1
  Selector2/1 -> [BackFadeGain]
  FadeIn/1 -> Delay6/1
  Bass Delay FR/1 -> Downsample/1
  Selector1/1 -> Expand Tail Components/1(Tail Comps)  "Ltail, Rtail, Ltail, Rtail"
  Bass/1 -> Bass Delay FR/1  "Lbass, Rbass"
  [BassDelayFull] -> Bass Delay FR/2
  [AlignmentDelay] -> Alignment Delay DR/2
  [BassDelayDec] -> Bass Delay DR/2
  Downsample/1 -> Bass Delay DR/1
  DRComps/1 -> Selector1/1, Alignment Delay DR/1
  Delay Tuning/1(Out1) -> [BassDelayDec]
  Delay Tuning/2(Out2) -> [BassDelayFull]
  Delay Tuning/3(Out3) -> [AlignmentDelay]
  VLS Gains Computation/1(D gains) -> D gains/1
  VLS Gains Computation/2(P gains) -> P gains/1
  Bass Delay DR/1 -> Premix/1(Bass In)  "Lbass, Rbass"
  Expand Tail Components/1(Wiggle Comps) -> Premix/3(Wiggle In)  "Lftail, Rftail, Lrtail, Rrtail"
  Premix/1(Out1) -> PremixOut/1
  FRComps/1 -> Full-rate Mixer/1(Upmix In)  "Lo, Ro, Limp, Ltail, Rimp, Rtail"
  Full-rate Mixer/1(Out1) -> FRMixerOut/1
  CAE Enable/1 -> Variant Source/2
  Constant3/1 -> Variant Source/1
  Variant Source/1 -> Premix/4(CAE Control), Full-rate Mixer/2(CAE Control)
  Alignment Delay DR/1 -> Premix/2(Upmix In)  "Lo, Ro, Ls, Rs, Limp, Ltail, Rimp, Rtail"

== system medusa5h1_stereo/Medusa + Holigram/Medusa5H1 Part 3/PremixCompSplitter ==
  note: Select Headrest Premix components
  note: Reorder as Non-headrest followed by Headrest speakers
  note: Select Peripheral Premix components
  note: Select Overhead Premix components
  PremixIn : Inport
  FRMixerIn : Inport  Port=2
  Selector : Selector  NumberOfDimensions=2  InputPortWidth=3  IndexOptions=Select all,Index vector (dialog)  Indices=[1 3],config.PeripheralIdx  OutputSizes=1,1
  Selector1 : Selector  NumberOfDimensions=2  InputPortWidth=3  IndexOptions=Select all,Index vector (dialog)  Indices=[1 3],config.HeadrestIdx  OutputSizes=1,1
  Selector2 : Selector  NumberOfDimensions=2  InputPortWidth=3  IndexOptions=Select all,Index vector (dialog)  Indices=[1 3],config.OverheadIdx  OutputSizes=1,1
  Selector4 : Selector  NumberOfDimensions=2  InputPortWidth=3  IndexOptions=Select all,Index vector (dialog)  Indices=[1 3],config.FRMOutputIdx  OutputSizes=1,1
  PeripheralPremixOut : Outport
  OverheadPremixOut : Outport  Port=2
  HeadrestPremixOut : Outport  Port=3
  FRMixerOut : Outport  Port=4
  wires:
  PremixIn/1 -> Selector1/1, Selector2/1, Selector/1
  Selector2/1 -> OverheadPremixOut/1
  Selector/1 -> PeripheralPremixOut/1
  Selector1/1 -> HeadrestPremixOut/1  "Lo, Ro, Ls, Rs, Lsr, Rsr"
  Selector4/1 -> FRMixerOut/1
  FRMixerIn/1 -> Selector4/1

== system medusa5h1_stereo/Medusa + Holigram/Medusa5H1 Part 4/Bypass ==
  Action Port : ActionPort
  Constant : Constant  Value=zeros(ConfigBTC.DeciRateFrameSize, ConfigBTC.NumPeripheralChannels)  OutDataTypeStr=single
  Constant1 : Constant  Value=zeros(ConfigBTC.DeciRateFrameSize, 2*ConfigBTC.NumHeadrestComps)  OutDataTypeStr=single
  Constant2 : Constant  Value=ConfigBTC.DefaultFullRateMixerOutput  OutDataTypeStr=single
  PeripheralOut : Outport  VectorParamsAs1DForOutWhenUnconnected=off
  HeadrestOut : Outport  Port=2  VectorParamsAs1DForOutWhenUnconnected=off
  FROut : Outport  Port=3  VectorParamsAs1DForOutWhenUnconnected=off
  wires:
  Constant/1 -> PeripheralOut/1
  Constant1/1 -> HeadrestOut/1
  Constant2/1 -> FROut/1

== system medusa5h1_stereo/Medusa + Holigram/Medusa5H1 Part 4/Enable State Write ==
  Trigger : TriggerPort  TriggerType=function-call  VariantControl=Variant  PortDimensions=1
  Constant : Constant  Value=0  OutDataTypeStr=uint32
  Data Store Write : DataStoreWrite  DataStoreName=MedusaHoligramEnable  IndexOptions=Index vector (dialog)  Indices=1  OutputSizes=1
  wires:
  Constant/1 -> Data Store Write/1

== system medusa5h1_stereo/Medusa + Holigram/Medusa5H1 Part 4/On ==
  PeripheralPremixOut : Inport  OutDataTypeStr=single
  HeadrestPremixOut : Inport  Port=2
  FRMixerOut : Inport  Port=3  OutDataTypeStr=single
  Action Port : ActionPort
  DR Mix Matrix with Hybrid Holigram EQ : MedusaDrHoligramEq/MedusaDrHoligramEq  Config=ConfigBTC.PeripheralHoligramEq.HoligramEq
  FR IIR Holigram EQ : MedusaFRHoligramEQ/FR Holigram EQ  configStruct=config.HoligramEQConfig
  Headrest Comp EQ : HeadrestCompEQ/Headrest Comp EQ  configStruct=vlsConfigStruct.HeadrestCompEQConfig
  PeripheralOut : Outport  VectorParamsAs1DForOutWhenUnconnected=off
  HeadrestOut : Outport  Port=2  VectorParamsAs1DForOutWhenUnconnected=off
  FROut : Outport  Port=3
  wires:
  HeadrestPremixOut/1 -> Headrest Comp EQ/1
  PeripheralPremixOut/1 -> DR Mix Matrix with Hybrid Holigram EQ/1
  FRMixerOut/1 -> FR IIR Holigram EQ/1
  FR IIR Holigram EQ/1 -> FROut/1
  Headrest Comp EQ/1 -> HeadrestOut/1
  DR Mix Matrix with Hybrid Holigram EQ/1 -> PeripheralOut/1

== system medusa5h1_stereo/Medusa + Holigram/Medusa5H1 Part 5/Bypass ==
  Action Port : ActionPort
  Constant : Constant  Value=zeros(ConfigBTC.DeciRateFrameSize, ConfigBTC.NumDeciRateChannels)  OutDataTypeStr=single
  Constant1 : Constant  Value=ConfigBTC.DefaultFullRateMixerOutput  OutDataTypeStr=single
  DRBypass : Outport  VectorParamsAs1DForOutWhenUnconnected=off
  FRBypass : Outport  Port=2  VectorParamsAs1DForOutWhenUnconnected=off
  wires:
  Constant/1 -> DRBypass/1
  Constant1/1 -> FRBypass/1

== system medusa5h1_stereo/Medusa + Holigram/Medusa5H1 Part 5/On ==
  PeripheralComps : Inport
  OverheadPremixOut : Inport  Port=2  OutDataTypeStr=single
  HeadrestComps : Inport  Port=3
  FRMixerOut : Inport  Port=4
  Action Port : ActionPort
  Gain : Gain
  Matrix Concatenate : Concatenate  NumInputs=3  Mode=Multidimensional array  ConcatenateDimension=2
  Overhead Holigram EQ : Subsystem  Variant=on
  Selector : Selector  NumberOfDimensions=2  InputPortWidth=3  IndexOptions=Select all,Index vector (dialog)  Indices=[1 3],config.holigramOutputSelect  OutputSizes=1,1
  DROut : Outport
  FROut : Outport  Port=2
  wires:
  OverheadPremixOut/1 -> Gain/1
  Gain/1 -> Overhead Holigram EQ/1(OH Comp In)
  Matrix Concatenate/1 -> Selector/1
  FRMixerOut/1 -> FROut/1
  Overhead Holigram EQ/1(Channels Out) -> Matrix Concatenate/2
  PeripheralComps/1 -> Matrix Concatenate/1
  HeadrestComps/1 -> Matrix Concatenate/3
  Selector/1 -> DROut/1
